simulink model "blk_learn"  (R2017a)
settings: Solver=VariableStepAuto  StartTime=0.0  StopTime=40  MaxStep=1e-3  RelTol=1e-3
libraries: truetime x1
settings Model: Creator=erich  LastModifiedBy=erich

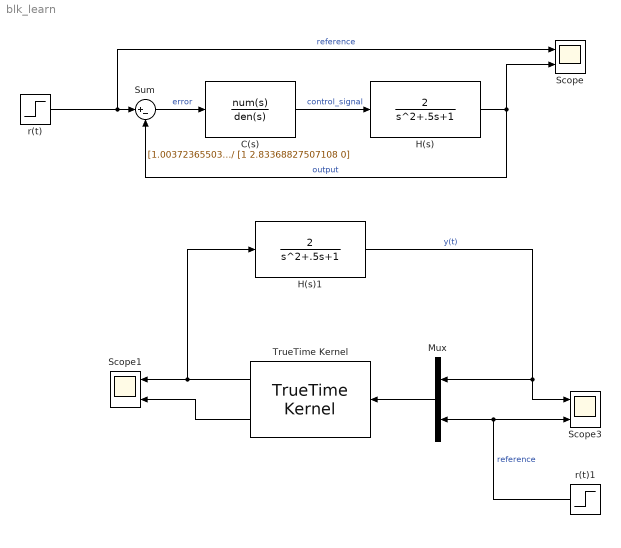
== system blk_learn ==
  C(s) : TransferFcn  Numerator=[1.00372365503441 0.501861827517207 1.00372365503441]  Denominator=[1 2.83368827507108 0]
  H(s) : TransferFcn  Numerator=[2]  Denominator=[1 .5 1]
  H(s)1 : TransferFcn  Numerator=[2]  Denominator=[1 .5 1]
  Mux : Mux  Inputs=2
  Scope : Scope  NumInputPorts=2
  Scope1 : Scope  NumInputPorts=2
  Scope3 : Scope  NumInputPorts=2
  Sum : Sum  Inputs=|+-
  TrueTime Kernel : truetime/TrueTime Kernel  sfun=init_cont  args=[]  ninputsoutputs=[2 1]  ntriggers=0  trigtype=falling  nwnodenbr=[]  clockoffsetdrift=[0 0]  schedoutput=on  battery=off  poweroutput=off
  r(t) : Step  SampleTime=0
  r(t)1 : Step  SampleTime=0
  wires:
  r(t)/1 -> Scope/1, Sum/1  "reference"
  H(s)/1 -> Scope/2, Sum/2  "output"
  Sum/1 -> C(s)/1  "error"
  C(s)/1 -> H(s)/1  "control_signal"
  TrueTime Kernel/1 -> Scope1/1, H(s)1/1
  Mux/1 -> TrueTime Kernel/1
  r(t)1/1 -> Mux/2, Scope3/2  "reference"
  H(s)1/1 -> Scope3/1, Mux/1  "y(t)"
  TrueTime Kernel/2 -> Scope1/2
